simulink model "MC31pwm"  (R2019a)
settings: Solver=ode23tb  StartTime=0.0  StopTime=0.08  RelTol=1e-3
libraries: powerlib x18
settings Model: Creator=z  LastModifiedBy=z
settings SolverCC: ZeroCrossAlgorithm=Adaptive
settings DataIOCC: ReturnWorkspaceOutputs=off
settings DebuggingCC: IgnoredZcDiagnostic=none  UnconnectedInputMsg=none  UnconnectedOutputMsg=none  UnconnectedLineMsg=none

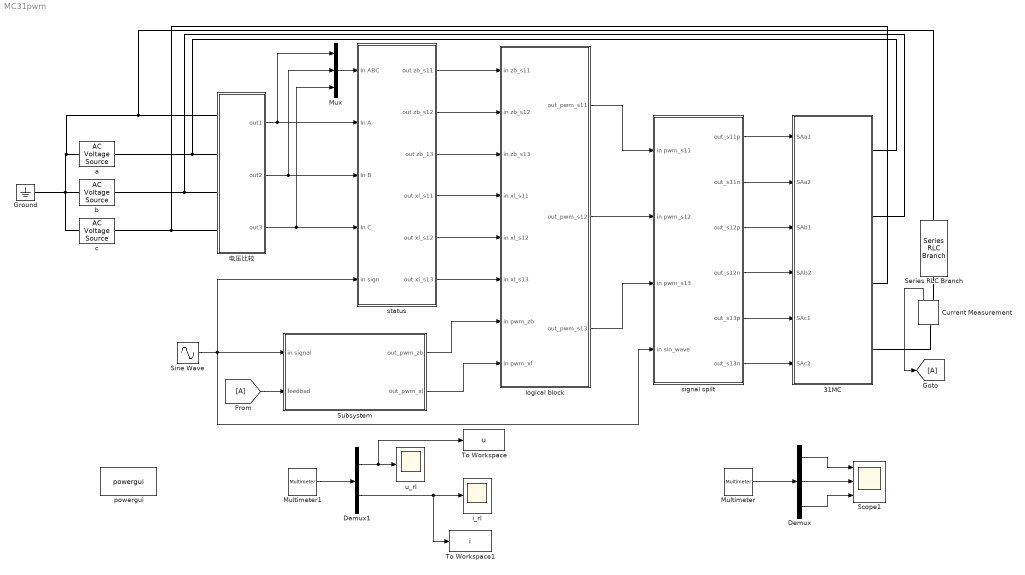
== system MC31pwm ==
  31MC : Subsystem
  Current Measurement : powerlib/Measurements/Current Measurement  PhasorSimulation=off  OutputType=Complex  PSBequivalent=0
      settings: SourceProductName=Simscape Electrical
  Demux : Demux  Outputs=3
  Demux1 : Demux  Outputs=2
  Ground : powerlib/Elements/Ground  LConnTagsString=a
      settings: SourceProductName=Simscape Electrical
  Multimeter : powerlib/Measurements/Multimeter  PhasorSimulation=off  OutputType=Complex  sel=[4 3 2]  L=5  Gain=[1 1 1]  yselected={'Usrc: a','Usrc: b','Usrc: c'};  PSBOutputType=1  PSBequivalent=0  AxesSetting=[0,0.1,-100,100]  Display=0  SavedBlockNames=-11
      settings: SourceProductName=Simscape Electrical
  Multimeter1 : powerlib/Measurements/Multimeter  PhasorSimulation=off  OutputType=Complex  sel=[1 5]  L=5  Gain=[1 1]  yselected={'Ub: Series RLC Branch','Ib: Series RLC Branch'};  PSBOutputType=1  PSBequivalent=0  AxesSetting=[0,0.1,-100,100]  Display=0  SavedBlockNames=-11
      settings: SourceProductName=Simscape Electrical
  Mux : Mux  Inputs=3
  Scope1 : Scope  NumInputPorts=3
  Series RLC Branch : powerlib/Elements/Series RLC Branch  LConnTagsString=__new0  RConnTagsString=__new0  BranchType=RL  Resistance=10  Inductance=0.01  SetiL0=off  InitialCurrent=0  Capacitance=1e-6  Setx0=off  InitialVoltage=0  Measurements=Branch voltage and current
      settings: SourceProductName=Simscape Electrical
  Sine Wave : Sin  Amplitude=10  Frequency=50*pi  SampleTime=0
  Subsystem : Subsystem
  To Workspace : ToWorkspace  VariableName=u  SaveFormat=Structure With Time  SampleTime=-1
  To Workspace1 : ToWorkspace  VariableName=i  SaveFormat=Structure With Time  SampleTime=-1
  a : powerlib/Electrical Sources/AC Voltage Source  Amplitude=220*sqrt(2)  Phase=0  Frequency=50  SampleTime=0  Measurements=Voltage  BusType=swing  Pref=10e3  Qref=0  Qmin=-inf  Qmax=+inf
      settings: SourceProductName=Simscape Electrical
  b : powerlib/Electrical Sources/AC Voltage Source  Amplitude=220*sqrt(2)  Phase=120  Frequency=50  SampleTime=0  Measurements=Voltage  BusType=swing  Pref=10e3  Qref=0  Qmin=-inf  Qmax=+inf
      settings: SourceProductName=Simscape Electrical
  c : powerlib/Electrical Sources/AC Voltage Source  Amplitude=220*sqrt(2)  Phase=240  Frequency=50  SampleTime=0  Measurements=Voltage  BusType=swing  Pref=10e3  Qref=0  Qmin=-inf  Qmax=+inf
      settings: SourceProductName=Simscape Electrical
  i_rl : Scope
  logical block : Subsystem
  powergui : powerlib/powergui  Priority=1  SimulationMode=Continuous  SampleTime=50e-6  frequency=60  Iterations=50  frequencyindice=50  Pbase=100e6  ErrMax=1e-4  UnitsV=kV  UnitsW=MW  buscounter=0  FunctionMessages=off  echomessages=off  EnableUseOfTLC=off  CurrentSourceSwitches=off  DisableSnubberDevices=off  DisableRonSwitches=off  DisableVfSwitches=off  DisplayEquations=off  AutomaticDiscreteSolvers=off  SolverType=Tustin/Backward Euler (TBE)  Interpol=off  ExternalGateDelay=off  methode=off  Ts=100  x0status=blocks  SPID=on  SwTol=0  HookPort=off  NonlinearTolerance=0  nMaxIteration=15  ContinueOnMaxIteration=off  RestoreLinks=warning  ResistiveCurrentMeasurement=off  Frange=[0:2:500]  Ylog=off  Xlog=on  ShowGrid=off  save=off  variable=ZData  structure=i  ZoomFFT=off  StartTime=0.0  cycles=1  DisplayStyle=1  fundamental=25  FreqAxis=off  MaxFrequency=1000  frequencyindicesteady=1  RmsSteady=1  display=off
      settings: SourceProductName=Simscape Electrical
  signal spilt : Subsystem
  status : Subsystem
  u_rl : Scope
  电压比较 : Subsystem
  wires:
  电压比较/1(out1) -> Mux/1, status/2(In A)
  电压比较/2(out2) -> Mux/2, status/3(In B)
  Mux/1 -> status/1(In ABC)
  电压比较/3(out3) -> Mux/3, status/4(In C)
  status/1(out zb_s11) -> logical block/1(in zb_s11)
  status/2(out zb_s12) -> logical block/2(in zb_s12)
  status/3(out zb_13) -> logical block/3(in zb_s13)
  status/5(out xl_s12) -> logical block/5(in xl_s12)
  logical block/2(out_pwm_s12) -> signal spilt/2(in pwm_s12)
  logical block/1(out_pwm_s11) -> signal spilt/1(in pwm_s11)
  logical block/3(out_pwm_s13) -> signal spilt/3(in pwm_s13)
  status/4(out xl_s11) -> logical block/4(in xl_s11)
  status/6(out xl_s13) -> logical block/6(in xl_s13)
  signal spilt/1(out_s11p) -> 31MC/1(SAa1)
  signal spilt/2(out_s11n) -> 31MC/2(SAa2)
  signal spilt/3(out_s12p) -> 31MC/3(SAb1)
  signal spilt/4(out_s12n) -> 31MC/4(SAb2)
  signal spilt/5(out_s13p) -> 31MC/5(SAc1)
  signal spilt/6(out_s13n) -> 31MC/6(SAc2)
  Subsystem/1(out_pwm_zb) -> logical block/7(in pwm_zb)
  Current Measurement/1 -> [A]
  [A] -> Subsystem/2(feedbad)
  Sine Wave/1 -> status/5(in sign), signal spilt/4(in sin_wave), Subsystem/1(in signal)
  Demux/2 -> Scope1/2
  Demux/1 -> Scope1/1
  Demux/3 -> Scope1/3
  Multimeter/1 -> Demux/1
  Demux1/1 -> To Workspace/1, u_rl/1
  Multimeter1/1 -> Demux1/1
  Demux1/2 -> To Workspace1/1, i_rl/1
  Subsystem/2(out_pwm_xl) -> logical block/8(in pwm_xl)
  connections:
  31MC/RConn1 -- 电压比较/LConn2 -- a/RConn1
  31MC/RConn2 -- b/RConn1 -- 电压比较/LConn3
  31MC/RConn3 -- 电压比较/LConn4 -- c/RConn1
  Ground/LConn1 -- Series RLC Branch/RConn1 -- 电压比较/LConn1 -- a/LConn1 -- c/LConn1 -- b/LConn1
  Current Measurement/RConn1 -- Series RLC Branch/LConn1
  Current Measurement/LConn1 -- 31MC/RConn4

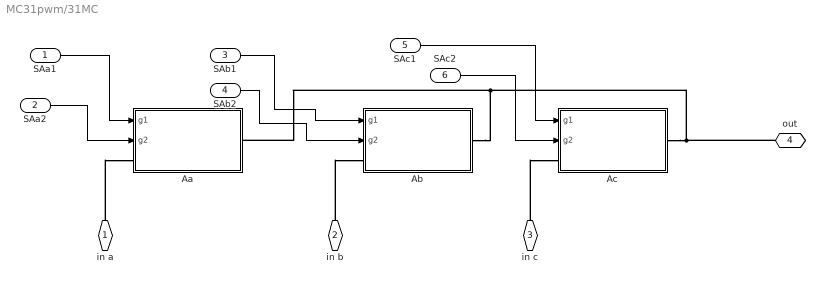
== system MC31pwm/31MC ==
  SAa1 : Inport
  SAa2 : Inport  Port=2
  SAb1 : Inport  Port=3
  SAb2 : Inport  Port=4
  SAc1 : Inport  Port=5
  SAc2 : Inport  Port=6
  Aa : Subsystem
  Ab : Subsystem
  Ac : Subsystem
  in a : PMIOPort  Side=Right
  in b : PMIOPort  Port=2  Side=Right
  in c : PMIOPort  Port=3  Side=Right
  out : PMIOPort  Port=4  Side=Right
  wires:
  SAb1/1 -> Ab/1(g1)
  SAa2/1 -> Aa/2(g2)
  SAb2/1 -> Ab/2(g2)
  SAc2/1 -> Ac/2(g2)
  SAc1/1 -> Ac/1(g1)
  SAa1/1 -> Aa/1("g1 ")
  connections:
  in b/RConn1 -- Ab/LConn1
  Ac/RConn1 -- out/RConn1 -- Aa/RConn1 -- Ab/RConn1
  in a/RConn1 -- Aa/LConn1
  in c/RConn1 -- Ac/LConn1

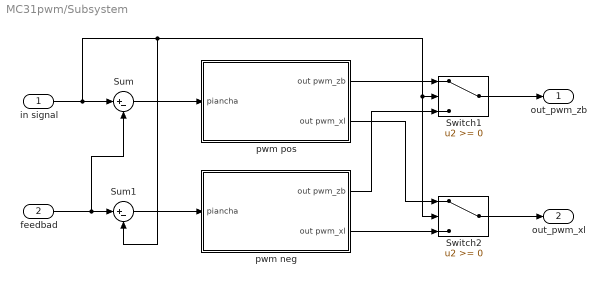
== system MC31pwm/Subsystem ==
  in signal : Inport
  feedbad : Inport  Port=2
  Sum : Sum  Inputs=|+-
  Sum1 : Sum  Inputs=|+-
  Switch1 : Switch
  Switch2 : Switch
  pwm neg : Subsystem
  pwm pos : Subsystem
  out_pwm_zb : Outport
  out_pwm_xl : Outport  Port=2
  wires:
  pwm pos/2(out pwm_xl) -> Switch2/1
  pwm pos/1(out pwm_zb) -> Switch1/1
  in signal/1 -> Sum1/2, Switch2/2, Switch1/2, Sum/1
  pwm neg/1(out pwm_zb) -> Switch1/3
  Sum/1 -> pwm pos/1(piancha)
  pwm neg/2(out pwm_xl) -> Switch2/3
  Switch1/1 -> out_pwm_zb/1
  feedbad/1 -> Sum/2, Sum1/1
  Sum1/1 -> pwm neg/1(piancha)
  Switch2/1 -> out_pwm_xl/1

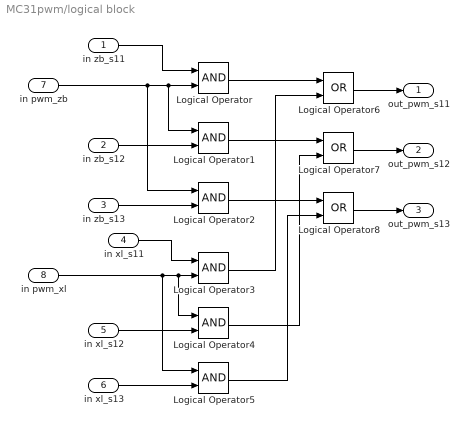
== system MC31pwm/logical block ==
  in zb_s11 : Inport
  in zb_s12 : Inport  Port=2
  in zb_s13 : Inport  Port=3
  in xl_s11 : Inport  Port=4
  in xl_s12 : Inport  Port=5
  in xl_s13 : Inport  Port=6
  in pwm_zb : Inport  Port=7
  in pwm_xl : Inport  Port=8
  Logical Operator{,1..5} (6 alike) : Logic  AllPortsSameDT=off  OutDataTypeStr=boolean
  Logical Operator6 : Logic  Operator=OR  AllPortsSameDT=off  OutDataTypeStr=boolean
  Logical Operator7 : Logic  Operator=OR  AllPortsSameDT=off  OutDataTypeStr=boolean
  Logical Operator8 : Logic  Operator=OR  AllPortsSameDT=off  OutDataTypeStr=boolean
  out_pwm_s11 : Outport
  out_pwm_s12 : Outport  Port=2
  out_pwm_s13 : Outport  Port=3
  wires:
  in pwm_xl/1 -> Logical Operator5/1, Logical Operator4/1, Logical Operator3/2
  in xl_s12/1 -> Logical Operator4/2
  Logical Operator4/1 -> Logical Operator7/2
  in xl_s13/1 -> Logical Operator5/2
  Logical Operator1/1 -> Logical Operator7/1
  Logical Operator2/1 -> Logical Operator8/1
  Logical Operator7/1 -> out_pwm_s12/1
  Logical Operator6/1 -> out_pwm_s11/1
  in zb_s12/1 -> Logical Operator1/2
  in xl_s11/1 -> Logical Operator3/1
  in zb_s13/1 -> Logical Operator2/2
  Logical Operator8/1 -> out_pwm_s13/1
  in pwm_zb/1 -> Logical Operator2/1, Logical Operator1/1, Logical Operator/2
  Logical Operator3/1 -> Logical Operator6/2
  in zb_s11/1 -> Logical Operator/1
  Logical Operator5/1 -> Logical Operator8/2
  Logical Operator/1 -> Logical Operator6/1

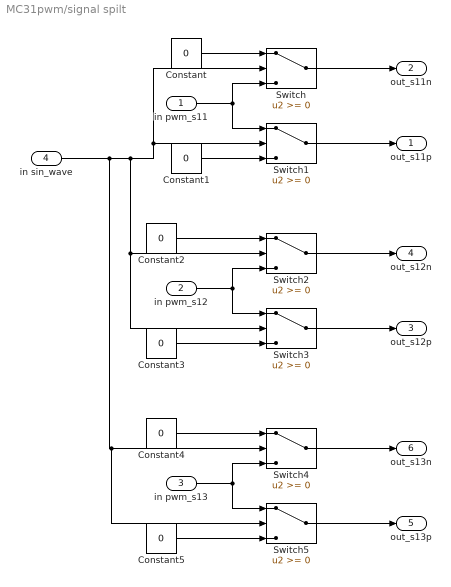
== system MC31pwm/signal spilt ==
  in pwm_s11 : Inport
  in pwm_s12 : Inport  Port=2
  in pwm_s13 : Inport  Port=3
  in sin_wave : Inport  Port=4
  Constant{,1..5} (6 alike) : Constant  Value=0
  Switch{,1..5} (6 alike) : Switch
  out_s11p : Outport
  out_s11n : Outport  Port=2
  out_s12p : Outport  Port=3
  out_s12n : Outport  Port=4
  out_s13p : Outport  Port=5
  out_s13n : Outport  Port=6
  wires:
  Switch3/1 -> out_s12p/1
  Constant/1 -> Switch/1
  Constant2/1 -> Switch2/1
  Switch5/1 -> out_s13p/1
  Switch1/1 -> out_s11p/1
  in sin_wave/1 -> Switch5/2, Switch4/2, Switch3/2, Switch2/2, Switch/2, Switch1/2
  in pwm_s12/1 -> Switch3/1, Switch2/3
  Constant1/1 -> Switch1/3
  in pwm_s13/1 -> Switch5/1, Switch4/3
  Switch2/1 -> out_s12n/1
  Switch4/1 -> out_s13n/1
  Constant3/1 -> Switch3/3
  Constant5/1 -> Switch5/3
  Switch/1 -> out_s11n/1
  in pwm_s11/1 -> Switch1/1, Switch/3
  Constant4/1 -> Switch4/1

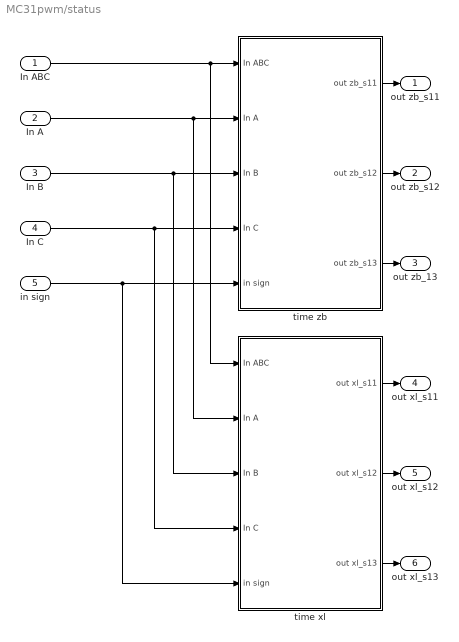
== system MC31pwm/status ==
  In ABC : Inport
  In A : Inport  Port=2
  In B : Inport  Port=3
  In C : Inport  Port=4
  in sign : Inport  Port=5
  time xl : Subsystem
  time zb : Subsystem
  out zb_s11 : Outport
  out zb_s12 : Outport  Port=2
  out zb_13 : Outport  Port=3
  out xl_s11 : Outport  Port=4
  out xl_s12 : Outport  Port=5
  out xl_s13 : Outport  Port=6
  wires:
  In B/1 -> time xl/3(In B), time zb/3(In B)
  in sign/1 -> time xl/5(in sign), time zb/5(in sign)
  In A/1 -> time xl/2(In A), time zb/2(In A)
  In ABC/1 -> time xl/1(In ABC), time zb/1(In ABC)
  time xl/1(out xl_s11) -> out xl_s11/1
  In C/1 -> time xl/4(In C), time zb/4(In C)
  time zb/1(out zb_s11) -> out zb_s11/1
  time xl/3(out xl_s13) -> out xl_s13/1
  time xl/2(out xl_s12) -> out xl_s12/1
  time zb/3(out zb_s13) -> out zb_13/1
  time zb/2(out zb_s12) -> out zb_s12/1

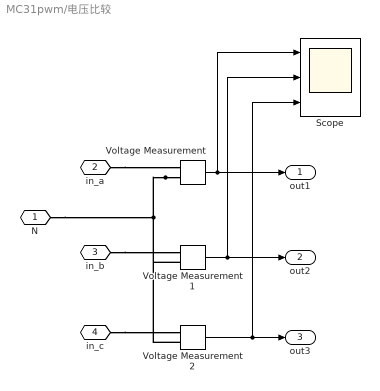
== system MC31pwm/电压比较 ==
  Scope : Scope  NumInputPorts=3
  Voltage Measurement : powerlib/Measurements/Voltage Measurement  PhasorSimulation=off  OutputType=Complex  PSBequivalent=0
      settings: SourceProductName=Simscape Electrical
  Voltage Measurement1 : powerlib/Measurements/Voltage Measurement  PhasorSimulation=off  OutputType=Complex  PSBequivalent=0
      settings: SourceProductName=Simscape Electrical
  Voltage Measurement2 : powerlib/Measurements/Voltage Measurement  PhasorSimulation=off  OutputType=Complex  PSBequivalent=0
      settings: SourceProductName=Simscape Electrical
  N : PMIOPort  Side=Left
  in_a : PMIOPort  Port=2  Side=Left
  in_b : PMIOPort  Port=3  Side=Left
  in_c : PMIOPort  Port=4  Side=Left
  out1 : Outport
  out2 : Outport  Port=2
  out3 : Outport  Port=3
  wires:
  Voltage Measurement2/1 -> Scope/3, out3/1
  Voltage Measurement/1 -> Scope/1, out1/1
  Voltage Measurement1/1 -> Scope/2, out2/1
  connections:
  in_a/RConn1 -- Voltage Measurement/LConn1
  Voltage Measurement/LConn2 -- N/RConn1 -- Voltage Measurement2/LConn2 -- Voltage Measurement1/LConn2
  in_b/RConn1 -- Voltage Measurement1/LConn1
  in_c/RConn1 -- Voltage Measurement2/LConn1

== system MC31pwm/31MC/Aa ==
  "g1 " : Inport
  g2 : Inport  Port=2
  IGBT/Diode : powerlib/Power Electronics/IGBT//Diode  Ron=1e-3  Rs=1e5  Cs=inf  Measurements=on
      settings: SourceProductName=Simscape Electrical
  IGBT/Diode1 : powerlib/Power Electronics/IGBT//Diode  Ron=1e-3  Rs=1e5  Cs=inf  Measurements=on
      settings: SourceProductName=Simscape Electrical
  Terminator : Terminator
  Terminator1 : Terminator
  1 : PMIOPort  Side=Left
  2 : PMIOPort  Port=2  Side=Right
  wires:
  IGBT/Diode1/1 -> Terminator/1
  "g1 "/1 -> IGBT/Diode/1
  IGBT/Diode/1 -> Terminator1/1
  g2/1 -> IGBT/Diode1/1
  connections:
  1/RConn1 -- IGBT/Diode/LConn1
  IGBT/Diode1/RConn1 -- IGBT/Diode/RConn1
  2/RConn1 -- IGBT/Diode1/LConn1

== system MC31pwm/31MC/Ab ==
  g1 : Inport
  g2 : Inport  Port=2
  IGBT/Diode : powerlib/Power Electronics/IGBT//Diode  Ron=1e-3  Rs=1e5  Cs=inf  Measurements=on
      settings: SourceProductName=Simscape Electrical
  IGBT/Diode1 : powerlib/Power Electronics/IGBT//Diode  Ron=1e-3  Rs=1e5  Cs=inf  Measurements=on
      settings: SourceProductName=Simscape Electrical
  Terminator : Terminator
  Terminator1 : Terminator
  1 : PMIOPort  Side=Left
  2 : PMIOPort  Port=2  Side=Right
  wires:
  IGBT/Diode1/1 -> Terminator/1
  g1/1 -> IGBT/Diode/1
  IGBT/Diode/1 -> Terminator1/1
  g2/1 -> IGBT/Diode1/1
  connections:
  1/RConn1 -- IGBT/Diode/LConn1
  IGBT/Diode1/RConn1 -- IGBT/Diode/RConn1
  2/RConn1 -- IGBT/Diode1/LConn1

== system MC31pwm/31MC/Ac ==
  g1 : Inport
  g2 : Inport  Port=2
  IGBT/Diode : powerlib/Power Electronics/IGBT//Diode  Ron=1e-3  Rs=1e5  Cs=inf  Measurements=on
      settings: SourceProductName=Simscape Electrical
  IGBT/Diode1 : powerlib/Power Electronics/IGBT//Diode  Ron=1e-3  Rs=1e5  Cs=inf  Measurements=on
      settings: SourceProductName=Simscape Electrical
  Terminator : Terminator
  Terminator1 : Terminator
  1 : PMIOPort  Side=Left
  2 : PMIOPort  Port=2  Side=Right
  wires:
  IGBT/Diode1/1 -> Terminator/1
  g1/1 -> IGBT/Diode/1
  IGBT/Diode/1 -> Terminator1/1
  g2/1 -> IGBT/Diode1/1
  connections:
  1/RConn1 -- IGBT/Diode/LConn1
  IGBT/Diode1/RConn1 -- IGBT/Diode/RConn1
  2/RConn1 -- IGBT/Diode1/LConn1

== system MC31pwm/Subsystem/pwm neg ==
  piancha : Inport
  Logical Operator : Logic  Operator=NOT  AllPortsSameDT=off  OutDataTypeStr=boolean
  Relay : Relay  OnSwitchValue=0.1
  out pwm_zb : Outport
  out pwm_xl : Outport  Port=2
  wires:
  Relay/1 -> out pwm_xl/1, Logical Operator/1
  piancha/1 -> Relay/1
  Logical Operator/1 -> out pwm_zb/1

== system MC31pwm/Subsystem/pwm pos ==
  piancha : Inport
  Logical Operator : Logic  Operator=NOT  AllPortsSameDT=off  OutDataTypeStr=boolean
  Relay : Relay  OnSwitchValue=0.1
  out pwm_zb : Outport
  out pwm_xl : Outport  Port=2
  wires:
  Logical Operator/1 -> out pwm_xl/1
  Relay/1 -> out pwm_zb/1, Logical Operator/1
  piancha/1 -> Relay/1

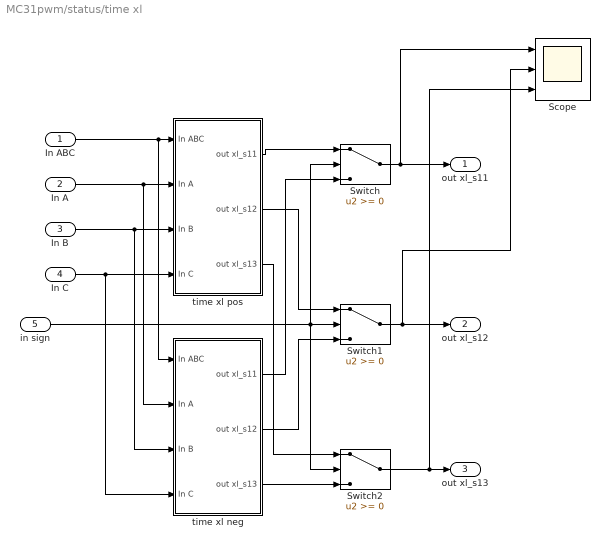
== system MC31pwm/status/time xl ==
  In ABC : Inport
  In A : Inport  Port=2
  In B : Inport  Port=3
  In C : Inport  Port=4
  in sign : Inport  Port=5
  Scope : Scope  NumInputPorts=3
  Switch : Switch
  Switch1 : Switch
  Switch2 : Switch
  time xl neg : Subsystem
  time xl pos : Subsystem
  out xl_s11 : Outport
  out xl_s12 : Outport  Port=2
  out xl_s13 : Outport  Port=3
  wires:
  in sign/1 -> Switch2/2, Switch/2, Switch1/2
  In B/1 -> time xl pos/3(In B), time xl neg/3(In B)
  In C/1 -> time xl pos/4(In C), time xl neg/4(In C)
  In A/1 -> time xl neg/2(In A), time xl pos/2(In A)
  time xl pos/3(out xl_s13) -> Switch2/1
  Switch2/1 -> Scope/3, out xl_s13/1
  time xl neg/3(out xl_s13) -> Switch2/3
  time xl neg/1(out xl_s11) -> Switch/3
  Switch1/1 -> Scope/2, out xl_s12/1
  In ABC/1 -> time xl pos/1(In ABC), time xl neg/1(In ABC)
  time xl neg/2(out xl_s12) -> Switch1/3
  time xl pos/2(out xl_s12) -> Switch1/1
  time xl pos/1(out xl_s11) -> Switch/1
  Switch/1 -> Scope/1, out xl_s11/1

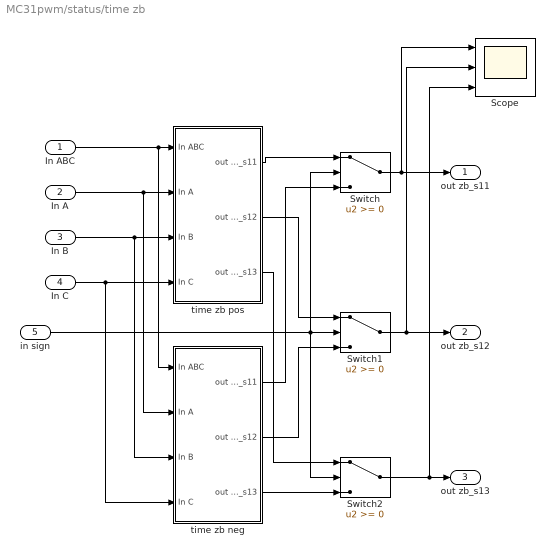
== system MC31pwm/status/time zb ==
  In ABC : Inport
  In A : Inport  Port=2
  In B : Inport  Port=3
  In C : Inport  Port=4
  in sign : Inport  Port=5
  Scope : Scope  NumInputPorts=3
  Switch : Switch
  Switch1 : Switch
  Switch2 : Switch
  time zb neg : Subsystem
  time zb pos : Subsystem
  out zb_s11 : Outport
  out zb_s12 : Outport  Port=2
  out zb_s13 : Outport  Port=3
  wires:
  in sign/1 -> Switch2/2, Switch/2, Switch1/2
  In B/1 -> time zb pos/3(In B), time zb neg/3(In B)
  In C/1 -> time zb pos/4(In C), time zb neg/4(In C)
  In A/1 -> time zb neg/2(In A), time zb pos/2(In A)
  time zb pos/3(out zb_s13) -> Switch2/1
  Switch2/1 -> Scope/3, out zb_s13/1
  time zb neg/3(out zb_s13) -> Switch2/3
  time zb neg/1(out zb_s11) -> Switch/3
  Switch1/1 -> Scope/2, out zb_s12/1
  In ABC/1 -> time zb pos/1(In ABC), time zb neg/1(In ABC)
  time zb neg/2(out zb_s12) -> Switch1/3
  time zb pos/2(out zb_s12) -> Switch1/1
  time zb pos/1(out zb_s11) -> Switch/1
  Switch/1 -> Scope/1, out zb_s11/1

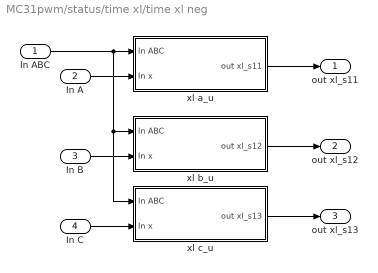
== system MC31pwm/status/time xl/time xl neg ==
  In ABC : Inport
  In A : Inport  Port=2
  In B : Inport  Port=3
  In C : Inport  Port=4
  xl a_u : Subsystem
  xl b_u : Subsystem
  xl c_u : Subsystem
  out xl_s11 : Outport
  out xl_s12 : Outport  Port=2
  out xl_s13 : Outport  Port=3
  wires:
  xl c_u/1(out xl_s13) -> out xl_s13/1
  In A/1 -> xl a_u/2(In x)
  xl b_u/1(out xl_s12) -> out xl_s12/1
  In B/1 -> xl b_u/2(In x)
  In C/1 -> xl c_u/2(In x)
  In ABC/1 -> xl c_u/1(In ABC), xl b_u/1(In ABC), xl a_u/1(In ABC)
  xl a_u/1(out xl_s11) -> out xl_s11/1

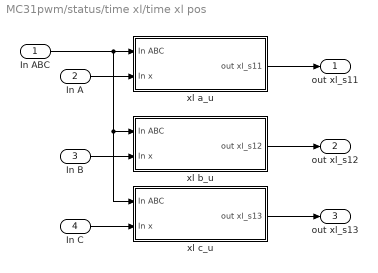
== system MC31pwm/status/time xl/time xl pos ==
  In ABC : Inport
  In A : Inport  Port=2
  In B : Inport  Port=3
  In C : Inport  Port=4
  xl a_u : Subsystem
  xl b_u : Subsystem
  xl c_u : Subsystem
  out xl_s11 : Outport
  out xl_s12 : Outport  Port=2
  out xl_s13 : Outport  Port=3
  wires:
  xl c_u/1(out xl_s13) -> out xl_s13/1
  In A/1 -> xl a_u/2(In x)
  xl b_u/1(out xl_s12) -> out xl_s12/1
  In B/1 -> xl b_u/2(In x)
  In C/1 -> xl c_u/2(In x)
  In ABC/1 -> xl c_u/1(In ABC), xl b_u/1(In ABC), xl a_u/1(In ABC)
  xl a_u/1(out xl_s11) -> out xl_s11/1

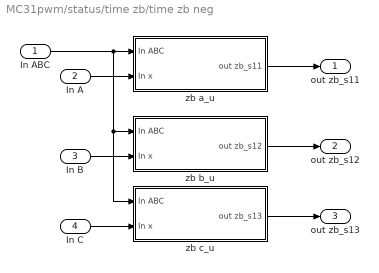
== system MC31pwm/status/time zb/time zb neg ==
  In ABC : Inport
  In A : Inport  Port=2
  In B : Inport  Port=3
  In C : Inport  Port=4
  zb a_u : Subsystem
  zb b_u : Subsystem
  zb c_u : Subsystem
  out zb_s11 : Outport
  out zb_s12 : Outport  Port=2
  out zb_s13 : Outport  Port=3
  wires:
  zb c_u/1(out zb_s13) -> out zb_s13/1
  In A/1 -> zb a_u/2(In x)
  zb b_u/1(out zb_s12) -> out zb_s12/1
  In B/1 -> zb b_u/2(In x)
  In C/1 -> zb c_u/2(In x)
  In ABC/1 -> zb c_u/1(In ABC), zb b_u/1(In ABC), zb a_u/1(In ABC)
  zb a_u/1(out zb_s11) -> out zb_s11/1

== system MC31pwm/status/time zb/time zb pos ==
  In ABC : Inport
  In A : Inport  Port=2
  In B : Inport  Port=3
  In C : Inport  Port=4
  zb a_u : Subsystem
  zb b_u : Subsystem
  zb c_u : Subsystem
  out zb_s11 : Outport
  out zb_s12 : Outport  Port=2
  out zb_s13 : Outport  Port=3
  wires:
  zb c_u/1(out zb_s13) -> out zb_s13/1
  In A/1 -> zb a_u/2(In x)
  zb b_u/1(out zb_s12) -> out zb_s12/1
  In B/1 -> zb b_u/2(In x)
  In C/1 -> zb c_u/2(In x)
  In ABC/1 -> zb c_u/1(In ABC), zb b_u/1(In ABC), zb a_u/1(In ABC)
  zb a_u/1(out zb_s11) -> out zb_s11/1

== system MC31pwm/status/time xl/time xl neg/xl a_u ==
  In ABC : Inport
  In x : Inport  Port=2
  Logical Operator : Logic  Operator=NOT  AllPortsSameDT=off  OutDataTypeStr=boolean
  MinMax : MinMax
  Sign : Signum
  Sum : Sum  Inputs=|+-
  out xl_s11 : Outport
  wires:
  MinMax/1 -> Sum/1
  In ABC/1 -> MinMax/1
  In x/1 -> Sum/2
  Sum/1 -> Sign/1
  Sign/1 -> Logical Operator/1
  Logical Operator/1 -> out xl_s11/1

== system MC31pwm/status/time xl/time xl neg/xl b_u ==
  In ABC : Inport
  In x : Inport  Port=2
  Logical Operator : Logic  Operator=NOT  AllPortsSameDT=off  OutDataTypeStr=boolean
  MinMax : MinMax
  Sign : Signum
  Sum : Sum  Inputs=|+-
  out xl_s12 : Outport
  wires:
  MinMax/1 -> Sum/1
  In ABC/1 -> MinMax/1
  In x/1 -> Sum/2
  Sum/1 -> Sign/1
  Logical Operator/1 -> out xl_s12/1
  Sign/1 -> Logical Operator/1

== system MC31pwm/status/time xl/time xl neg/xl c_u ==
  In ABC : Inport
  In x : Inport  Port=2
  Logical Operator : Logic  Operator=NOT  AllPortsSameDT=off  OutDataTypeStr=boolean
  MinMax : MinMax
  Sign : Signum
  Sum : Sum  Inputs=|+-
  out xl_s13 : Outport
  wires:
  MinMax/1 -> Sum/1
  In ABC/1 -> MinMax/1
  In x/1 -> Sum/2
  Sum/1 -> Sign/1
  Logical Operator/1 -> out xl_s13/1
  Sign/1 -> Logical Operator/1

== system MC31pwm/status/time xl/time xl pos/xl a_u ==
  In ABC : Inport
  In x : Inport  Port=2
  Logical Operator : Logic  Operator=NOT  AllPortsSameDT=off  OutDataTypeStr=boolean
  MinMax : MinMax
  Scope : Scope
  Sign : Signum
  Sum : Sum  Inputs=|+-
  out xl_s11 : Outport
  wires:
  Sign/1 -> Logical Operator/1
  MinMax/1 -> Sum/1
  Logical Operator/1 -> out xl_s11/1
  In ABC/1 -> MinMax/1
  In x/1 -> Sum/2
  Sum/1 -> Scope/1, Sign/1

== system MC31pwm/status/time xl/time xl pos/xl b_u ==
  In ABC : Inport
  In x : Inport  Port=2
  Logical Operator : Logic  Operator=NOT  AllPortsSameDT=off  OutDataTypeStr=boolean
  MinMax : MinMax
  Sign : Signum
  Sum : Sum  Inputs=|+-
  out xl_s12 : Outport
  wires:
  Sign/1 -> Logical Operator/1
  MinMax/1 -> Sum/1
  Logical Operator/1 -> out xl_s12/1
  In ABC/1 -> MinMax/1
  In x/1 -> Sum/2
  Sum/1 -> Sign/1

== system MC31pwm/status/time xl/time xl pos/xl c_u ==
  In ABC : Inport
  In x : Inport  Port=2
  Logical Operator : Logic  Operator=NOT  AllPortsSameDT=off  OutDataTypeStr=boolean
  MinMax : MinMax
  Sign : Signum
  Sum : Sum  Inputs=|+-
  out xl_s13 : Outport
  wires:
  Sign/1 -> Logical Operator/1
  MinMax/1 -> Sum/1
  Logical Operator/1 -> out xl_s13/1
  In ABC/1 -> MinMax/1
  In x/1 -> Sum/2
  Sum/1 -> Sign/1

== system MC31pwm/status/time zb/time zb neg/zb a_u ==
  In ABC : Inport
  In x : Inport  Port=2
  Logical Operator : Logic  Operator=NOT  AllPortsSameDT=off  OutDataTypeStr=boolean
  MinMax : MinMax  Function=max
  Sign : Signum
  Sum : Sum  Inputs=|+-
  out zb_s11 : Outport
  wires:
  MinMax/1 -> Sum/1
  In ABC/1 -> MinMax/1
  In x/1 -> Sum/2
  Sum/1 -> Sign/1
  Sign/1 -> Logical Operator/1
  Logical Operator/1 -> out zb_s11/1

== system MC31pwm/status/time zb/time zb neg/zb b_u ==
  In ABC : Inport
  In x : Inport  Port=2
  Logical Operator : Logic  Operator=NOT  AllPortsSameDT=off  OutDataTypeStr=boolean
  MinMax : MinMax  Function=max
  Sign : Signum
  Sum : Sum  Inputs=|+-
  out zb_s12 : Outport
  wires:
  MinMax/1 -> Sum/1
  In ABC/1 -> MinMax/1
  In x/1 -> Sum/2
  Sum/1 -> Sign/1
  Logical Operator/1 -> out zb_s12/1
  Sign/1 -> Logical Operator/1

== system MC31pwm/status/time zb/time zb neg/zb c_u ==
  In ABC : Inport
  In x : Inport  Port=2
  Logical Operator : Logic  Operator=NOT  AllPortsSameDT=off  OutDataTypeStr=boolean
  MinMax : MinMax  Function=max
  Sign : Signum
  Sum : Sum  Inputs=|+-
  out zb_s13 : Outport
  wires:
  MinMax/1 -> Sum/1
  In ABC/1 -> MinMax/1
  In x/1 -> Sum/2
  Sum/1 -> Sign/1
  Logical Operator/1 -> out zb_s13/1
  Sign/1 -> Logical Operator/1

== system MC31pwm/status/time zb/time zb pos/zb a_u ==
  In ABC : Inport
  In x : Inport  Port=2
  Logical Operator : Logic  Operator=NOT  AllPortsSameDT=off  OutDataTypeStr=boolean
  MinMax : MinMax  Function=max
  Scope : Scope
  Sign : Signum
  Sum : Sum  Inputs=|+-
  out zb_s11 : Outport
  wires:
  Sign/1 -> Logical Operator/1
  MinMax/1 -> Sum/1
  Logical Operator/1 -> out zb_s11/1
  In ABC/1 -> MinMax/1
  In x/1 -> Sum/2
  Sum/1 -> Scope/1, Sign/1

== system MC31pwm/status/time zb/time zb pos/zb b_u ==
  In ABC : Inport
  In x : Inport  Port=2
  Logical Operator : Logic  Operator=NOT  AllPortsSameDT=off  OutDataTypeStr=boolean
  MinMax : MinMax  Function=max
  Sign : Signum
  Sum : Sum  Inputs=|+-
  out zb_s12 : Outport
  wires:
  Sign/1 -> Logical Operator/1
  MinMax/1 -> Sum/1
  Logical Operator/1 -> out zb_s12/1
  In ABC/1 -> MinMax/1
  In x/1 -> Sum/2
  Sum/1 -> Sign/1

== system MC31pwm/status/time zb/time zb pos/zb c_u ==
  In ABC : Inport
  In x : Inport  Port=2
  Logical Operator : Logic  Operator=NOT  AllPortsSameDT=off  OutDataTypeStr=boolean
  MinMax : MinMax  Function=max
  Sign : Signum
  Sum : Sum  Inputs=|+-
  out zb_s13 : Outport
  wires:
  Sign/1 -> Logical Operator/1
  MinMax/1 -> Sum/1
  Logical Operator/1 -> out zb_s13/1
  In ABC/1 -> MinMax/1
  In x/1 -> Sum/2
  Sum/1 -> Sign/1
